simulink model "suspension-system-simulation"  (R2021b)
settings: Solver=VariableStepAuto  StartTime=0.0  StopTime=7  RelTol=1e-3
libraries: simulink x1
settings Model: Creator=nima8  LastModifiedBy=nima8

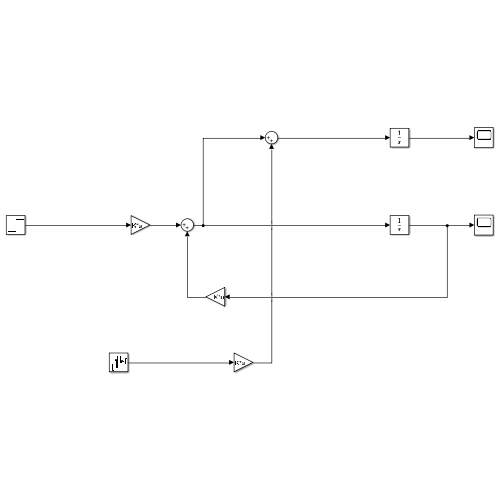
[thumbnail: Simulink's stored preview of the top-level diagram]
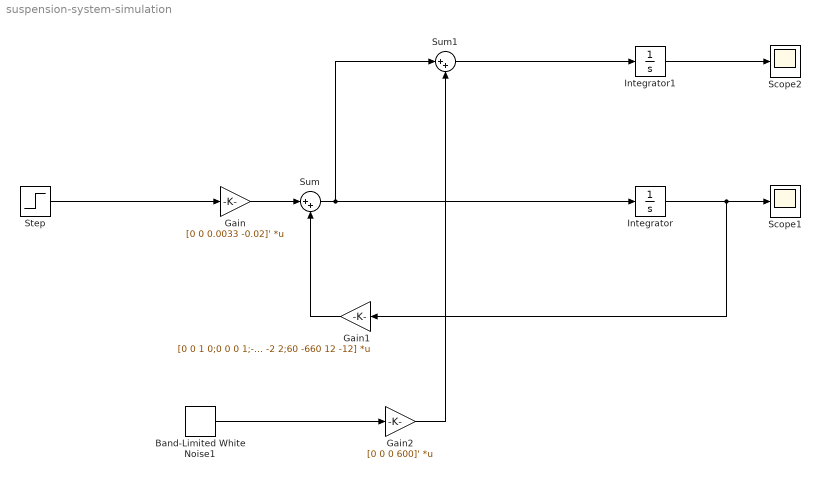
== system suspension-system-simulation ==
  Band-Limited White Noise1 : simulink/Sources/Band-Limited White Noise  Cov=[0.0001]  Ts=0.1  seed=[23341]
  Gain : Gain  Gain=[0 0 0.0033 -0.02]'  Multiplication=Matrix(K*u)
  Gain1 : Gain  Gain=[0 0 1 0;0 0 0 1;-10 10 -2 2;60 -660 12 -12]  Multiplication=Matrix(K*u)
  Gain2 : Gain  Gain=[0 0 0 600]'  Multiplication=Matrix(K*u)
  Integrator : Integrator  InitialCondition=[0.2 0 0 0]'
  Integrator1 : Integrator  InitialCondition=[0.2 0 0 0]'
  Scope1 : Scope
  Scope2 : Scope
  Step : Step  SampleTime=0
  Sum : Sum  Inputs=|++
  Sum1 : Sum  Inputs=|++
  wires:
  Step/1 -> Gain/1
  Gain/1 -> Sum/1
  Gain1/1 -> Sum/2
  Band-Limited White Noise1/1 -> Gain2/1
  Integrator/1 -> Scope1/1, Gain1/1
  Sum/1 -> Integrator/1, Sum1/1
  Gain2/1 -> Sum1/2
  Integrator1/1 -> Scope2/1
  Sum1/1 -> Integrator1/1
